simulink model "sistema_mecanico_lagrange_"  (R2013a)
settings: Solver=ode45  SolverMode=SingleTasking  StartTime=0.0  StopTime=2  RelTol=1e-3
settings Model: CovMetricSettings=dwe  CovHtmlReporting=off  covSaveCumulativeToWorkspaceVar=off  CovSaveSingleToWorkspaceVar=off  CovExternalEMLEnable=on  Creator=carma  LastModifiedBy=carma
settings DataIOCC: LimitDataPoints=off  SaveFormat=StructureWithTime
settings DebuggingCC: UnderspecifiedInitializationDetection=Simplified  MergeDetectMultiDrivingBlocksExec=error  SolverPrmCheckMsg=none  FrameProcessingCompatibilityMsg=error  StateNameClashWarn=none  SFUnexpectedBacktrackingDiag=error  SFNoUnconditionalDefaultTransitionDiag=error
settings HardwareCC: ProdBitPerPointer=64  ProdLargestAtomicFloat=Float  ProdIntDivRoundTo=Zero  ProdEndianess=LittleEndian  ProdHWDeviceType=Specified
settings ModelReferenceCC: PropagateSignalLabelsOutOfModel=on
settings GRTTargetCC: CodeReplacementLibrary=C99 (ISO)  GeneratePreprocessorConditionals=Use local settings

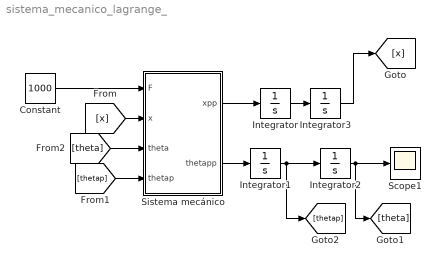
== system sistema_mecanico_lagrange_ ==
  Constant : Constant  Value=1000
  Integrator{,1..3} (4 alike) : Integrator
  Scope1 : Scope
      settings: TimeRange=auto  MaxDataPoints=5000  SaveToWorkspace=off  YMin=-0.12415  YMax=1.11739  SampleTime=-1
  Sistema mecánico : MATLAB Function  TreatAsAtomicUnit=on
      settings: PermitHierarchicalResolution=ParametersOnly
  wires:
  Constant/1 -> Sistema mecánico/1(F)
  Sistema mecánico/1(xpp) -> Integrator/1
  Sistema mecánico/2(thetapp) -> Integrator1/1
  Integrator1/1 -> [thetap], Integrator2/1
  Integrator/1 -> Integrator3/1
  Integrator3/1 -> [x]
  [x] -> Sistema mecánico/2(x)
  Integrator2/1 -> [theta], Scope1/1
  [thetap] -> Sistema mecánico/4(thetap)
  [theta] -> Sistema mecánico/3(theta)

== matlab function sistema_mecanico_lagrange_/Sistema mecánico ==
  data: F input; xpp output; x input; theta input; thetap input; thetapp output
function [xpp,thetapp] = fcn(F,x,theta, thetap)

%Parametros oscilaciones
r=0.01;
M=10;
k1=15;
k2=25;
k=10;
J=0.1;
b=2;



%ecuaciones dinámicas
xpp=(-k1*x-k2*(x-r*theta))/M;
thetapp=(F*r-k*theta-k2*r*(r*theta-x)-b*thetap)/J;
